simulink model "chi_square_simulation"  (Simulink 7.8)
settings: Solver=ode45  StartTime=0.0  StopTime=10.0  RelTol=1e-3
undefined symbols (not defined in the file): chitab, E, O
libraries: simulink x2
settings Model: Creator=Windows  LastModifiedBy=Windows
settings RTWCC: TargetLang=C++

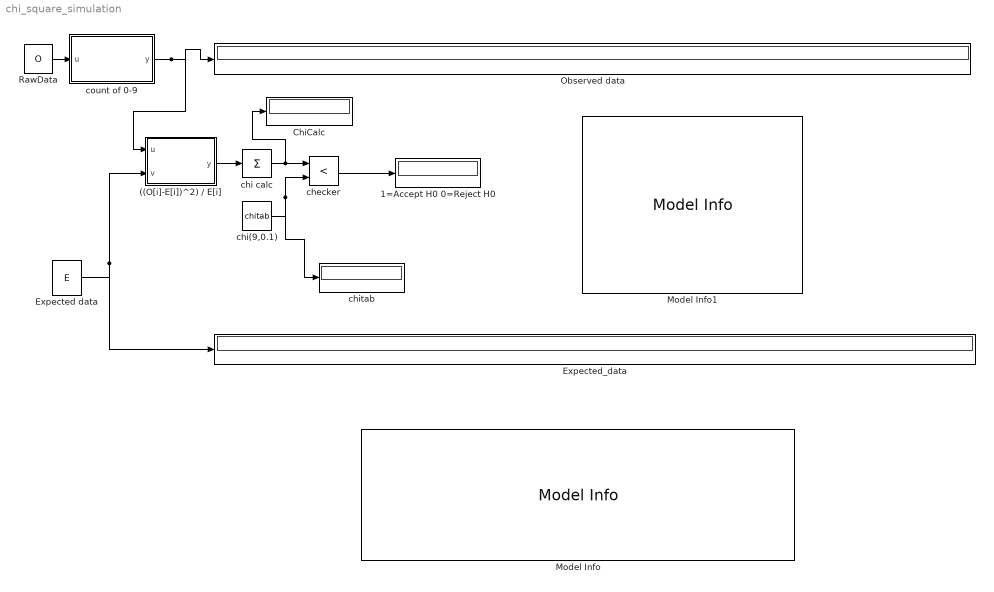
== system chi_square_simulation ==
  ((O[i]-E[i])^2) / E[i] : MATLAB Function  TreatAsAtomicUnit=on
  1=Accept H0 0=Reject H0 : Display
  ChiCalc : Display
  Expected data : Constant  Value=E
  Expected_data : Display
  Model Info : simulink/Model-Wide Utilities/Model Info  InitialBlockCM=None  BlockCM=None  Frame=on  DisplayStringWithTags=|  HorizontalTextAlignment=Center  LeftAlignmentValue=0.5  SourceBlockDiagram=chi_square_simulation  TagMaxNumber=20
      | Model Info
      | %<ModelName>
      | %<Created>
      | %<Description>This model helps in simulating chi-square test of random variable.
      | The model takes the observed data and expected data from user.
      | The model takes tabulated chi-square value from user.
      | The model gives appropriate decision based on test statistic result.
      | %<LastModificationDate>
  Model Info1 : simulink/Model-Wide Utilities/Model Info  InitialBlockCM=None  BlockCM=None  Frame=on  DisplayStringWithTags=|  HorizontalTextAlignment=Left  LeftAlignmentValue=0.02  SourceBlockDiagram=chi_square_simulation  TagMaxNumber=20
      | ************** Sample Raw Data***************
      |     O=[6,4,5,1,1,6,6,4,5,3,...
      |     	     7,0,6,4,0,9,0,0,6,9,...
      |     	     0,8,0,9,4,7,5,8,0,5,...
      |     	     6,2,4,8,7,7,8,1,6,4,...
      |     	     9,6,7,6,9,5,2,7,0,3,...
      |     	     9,6,1,0,2,4,5,0,6,8,...
      |     	     0,1,3,9,0,2,8,0,9,3,...
      |     	     6,2,5,6,1,3,8,6,7,3,...
      |     	     4,6,0,6,4,3,3,2,0,2,...
      |     	     6,8,7,7,8,3,1,8,0,4];
      |             E=[10,10,10,10,10,10,10,10,10,10];
      |             chitab=14.68
  Observed data : Display
  RawData : Constant  Value=O
  checker : RelationalOperator  Operator=<  OutDataTypeStr=boolean
  chi calc : Sum  Inputs=+
  chi(9,0.1) : Constant  Value=chitab
  chitab : Display
  count of 0-9 : MATLAB Function  TreatAsAtomicUnit=on
  wires:
  ((O[i]-E[i])^2) / E[i]/1(y) -> chi calc/1
  chi calc/1 -> checker/1, ChiCalc/1
  chi(9,0.1)/1 -> checker/2, chitab/1
  checker/1 -> 1=Accept H0 0=Reject H0/1
  Expected data/1 -> ((O[i]-E[i])^2) / E[i]/2(v), Expected_data/1
  RawData/1 -> count of 0-9/1(u)
  count of 0-9/1(y) -> ((O[i]-E[i])^2) / E[i]/1(u), Observed data/1

== matlab function count of 0-9 ==
  data: u input double; y output double
function y = count_of_rawdata(u)
%#codegen
O = zeros(1,10);
for k=1:1:10
    cnt=0;
    for l=1:1:length(u)
        if (k-1)==u(l)
            cnt=cnt+1;
        end
    end
    O(k)=cnt;
end
y = O;

== matlab function ((O[i]-E[i])^2) / E[i] ==
  data: u input double; y output double; v input double
function y = calculator(u,v)
%#codegen
O = zeros(1,length(u));
for ind=1:1:length(u)
    O(ind)=((u(ind)-v(ind))^2)/v(ind);
end
y=O;
